simulink model "inerziale"  (R2020b)
settings: Solver=FixedStepDiscrete  StartTime=0.0  StopTime=Inf  FixedStep=0.02  RelTol=1e-3  EnableMultiTasking=on
PostLoadFcn:
  | , if any(exist('dsrtsu_mdlpostloadfcn', 'file') == [2, 3, 6]), try dsrtsu_mdlpostloadfcn('Execute', bdroot); catch fprintf('Error in PostLoadFcn (dsrtsu_mdlpostloadfcn) for model "%s":\n %s\n', bdroot, lasterr); end, end,
settings Model: DSRTSU_INTERNAL_RTI_VER=470  DSRTSU_INTERNAL_RTI_TYPE=rti1006  SimulationMode=external  ExtModeTrigDuration=2  Creator=lapis_dspace  LastModifiedBy=ricca
settings DataIOCC: LimitDataPoints=on  ReturnWorkspaceOutputs=off
settings OptimizationCC: BlockReduction=off  OptimizeBlockIOStorage=off  BufferReuse=off  GlobalBufferReuse=off  ExpressionFolding=off  LocalBlockOutputs=off  LifeSpan=Inf  MaxStackSize=64  EfficientTunableParamExpr=on
settings DebuggingCC: AllowSymbolicDim=off  SFUnexpectedBacktrackingDiag=warning  SFNoUnconditionalDefaultTransitionDiag=warning  SFExecutionAtInitializationDiag=none  ArithmeticOperatorsInVariantConditions=warning
settings HardwareCC: ProdBitPerPointer=32  ProdBitPerSizeT=32  ProdBitPerPtrDiffT=32  ProdLargestAtomicInteger=Long  ProdLargestAtomicFloat=Double  ProdWordSize=32  ProdHWDeviceType=ARM Compatible->ARM Cortex  TargetIntDivRoundTo=Zero  TargetEndianess=LittleEndian  TargetHWDeviceType=Custom Processor->Custom  UseEmbeddedCoderFeatures=off  UseSimulinkCoderFeatures=off
settings ModelReferenceCC: PropagateSignalLabelsOutOfModel=off
settings SFSimCC: SimUseLocalCustomCode=off  MATLABDynamicMemAlloc=off  CustomCodeUndefinedFunction=UseInterfaceOnly
settings RTWCC: Description=Embedded Coder  SystemTargetFile=ert.tlc  HardwareBoard=Arduino Due  TemplateMakefile=ert_default_tmf  RTWUseLocalCustomCode=off  Toolchain=Arduino ARM  BuildConfiguration=Faster Runs
settings CodeAppCC: IgnoreCustomStorageClasses=off  MangleLength=10  StateflowObjectComments=on
settings ERTTargetCC: MultiwordLength=2048  SupportContinuousTime=on  SupportNonInlinedSFcns=on  SupportVariableSizeSignals=on  ConvertIfToSwitch=off  SuppressUnreachableDefaultCases=off
settings ConfigComp: CovMetricSettings=dw  CovSaveCumulativeToWorkspaceVar=on  CovSaveSingleToWorkspaceVar=on  CovExternalEMLEnable=off

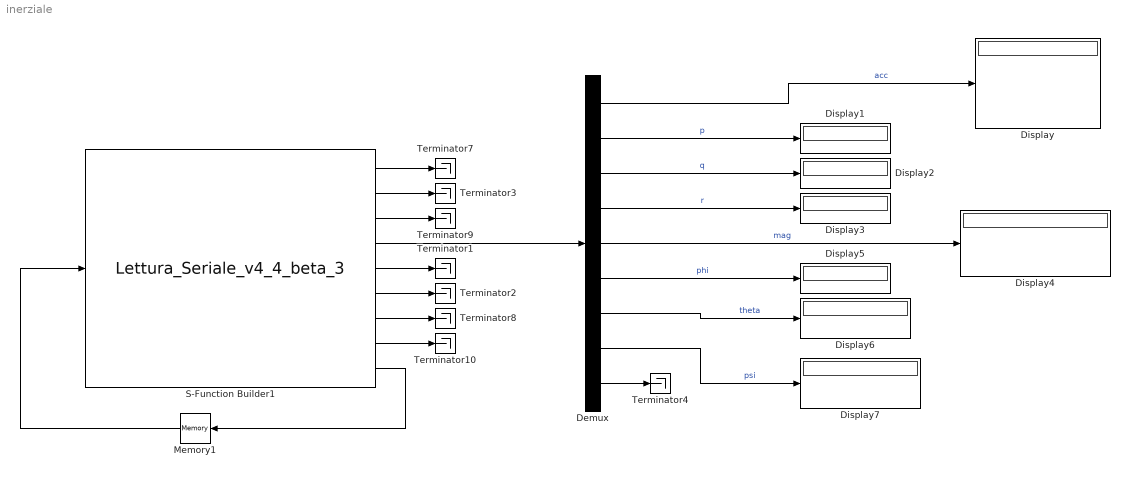
== system inerziale ==
  Demux : Demux  Outputs=[3 1 1 1 3 1 1 1 -1]
  Display{,1..7} (8 alike) : Display
  Memory1 : Memory  InheritSampleTime=on
  S-Function Builder1 : S-Function  InitFcn=try, set_param(gcb,'FunctionName','Lettura_Seriale_v4_4_beta_3'), end  FunctionName=Lettura_Seriale_v4_4_beta_3  Parameters=int16(int16(3)),int32(int32(115200))  SFunctionModules=Lettura_Seriale_v4_4_beta_3_wrapper Utility  SFunctionDeploymentMode=off  EnableBusSupport=off  mask(S-Function Builder){}
      mask init:
      | val = [[.9  0.75 0.75 1 1 .9 .9 1]',[1 1 0.75 0.75 .9 .9 1 .9]'];try , sys = get_param(gcb,'SfunBuilderFcnName');if isempty(sys), sys = get_param(gcb,'FunctionName'); end,catch, sys = get_param(gcb,'FunctionName'); end
      settings: CopyFcn=set_param(gcbh,'LinkStatus','none')  PreSaveFcn=try, set_param(gcb,'FunctionName','Lettura_Seriale_v4_4_beta_3'), end  OpenFcn=sfunctionwizard(gcbh)
      mask Display:
      | plot(val(:,1),val(:,2))
      | disp(sys)
      | port_label('input',1,'block_state_in')
      | port_label('output',1,'dato')
      | port_label('output',2,'uart_buffer')
      | port_label('output',3,'check')
      | port_label('output',4,'data_out')
      | port_label('output',5,'flag')
      | port_label('output',6,'counter')
      | port_label('output',7,'led_test')
      | port_label('output',8,'led_test_due')
      | port_label('output',9,'block_state_out')
  Terminator{1..4,7..10} (8 alike) : Terminator
  wires:
  S-Function Builder1/4 -> Demux/1
  S-Function Builder1/1 -> Terminator7/1
  S-Function Builder1/3 -> Terminator9/1
  S-Function Builder1/9 -> Memory1/1
  Memory1/1 -> S-Function Builder1/1
  S-Function Builder1/7 -> Terminator8/1
  S-Function Builder1/8 -> Terminator10/1
  S-Function Builder1/6 -> Terminator2/1
  S-Function Builder1/5 -> Terminator1/1
  S-Function Builder1/2 -> Terminator3/1
  Demux/8 -> Display7/1  "psi"
  Demux/7 -> Display6/1  "theta"
  Demux/6 -> Display5/1  "phi"
  Demux/5 -> Display4/1  "mag"
  Demux/4 -> Display3/1  "r"
  Demux/3 -> Display2/1  "q"
  Demux/2 -> Display1/1  "p"
  Demux/9 -> Terminator4/1
  Demux/1 -> Display/1  "acc"
